simulink model "UAV"  (R2025b)
settings: Solver=ode3  StartTime=0.0  StopTime=inf  FixedStep=Sim.Ts_fisica  RelTol=1e-3
PostLoadFcn:
  | Init
InitFcn:
  | Init
model workspace (MAT data in the model file):
  Mass = 1
undefined symbols (not defined in the file): DiscIntNeverNeededParam, Drone, DWORK0, DWORK1, DWORK10, DWORK11, DWORK12, DWORK13, DWORK14, DWORK15, DWORK16, DWORK17, DWORK18, DWORK19, DWORK2, DWORK20, DWORK21, DWORK22, DWORK23, DWORK24, DWORK3, DWORK4, DWORK5, DWORK6, DWORK7, DWORK8, DWORK9, F, Light, MIL, Sim
libraries: simulink x35, slpidlib x11, vrlib x4, aerolibwind2 x2, sim3dlib x2, uavsim3dlib x2
(part 8 of 8)

== system UAV/Pilot Interface/SIM_Flightstick_HotasX56 /Command Acquisition/Subsystem ==
  In1 : Inport
  Dead Zone{,1..4} (5 alike) : DeadZone  LowerValue=-0.05  UpperValue=0.05
  Demux : Demux  Outputs=5
  Selector : Selector  InputPortWidth=5  IndexOptions=Index vector (dialog)  Indices=[1 2 3 4 5]  OutputSizes=1
  Zero-Order Hold : ZeroOrderHold  SampleTime=1/100
  Roll : Outport
  Pitch : Outport  Port=2
  Yaw : Outport  Port=3
  Cx : Outport  Port=4
  Cy : Outport  Port=5
  wires:
  Demux/5 -> Dead Zone4/1
  Demux/4 -> Dead Zone3/1
  Demux/2 -> Dead Zone1/1
  Demux/3 -> Dead Zone2/1
  Demux/1 -> Dead Zone/1
  In1/1 -> Zero-Order Hold/1
  Selector/1 -> Demux/1
  Zero-Order Hold/1 -> Selector/1
  Dead Zone/1 -> Roll/1
  Dead Zone1/1 -> Pitch/1
  Dead Zone2/1 -> Cx/1
  Dead Zone3/1 -> Cy/1
  Dead Zone4/1 -> Yaw/1

== system UAV/Pilot Interface/SIM_Flightstick_HotasX56 /Command Acquisition/Subsystem1 ==
  In1 : Inport
  Demux1 : Demux  Outputs=14
  Selector : Selector  InputPortWidth=17  IndexOptions=Index vector (dialog)  Indices=[1 2 3 4 5 6 7 8 9 10 11 12 13 14]  OutputSizes=1
  Zero-Order Hold1 : ZeroOrderHold  SampleTime=1/100
  Trigger : Outport
  A : Outport  Port=2
  B : Outport  Port=3
  "C " : Outport  Port=4
  "D " : Outport  Port=5
  Lever : Outport  Port=6
  H1U : Outport  Port=7
  H1R : Outport  Port=8
  H1D : Outport  Port=9
  H1L : Outport  Port=10
  H2U : Outport  Port=11
  H2R : Outport  Port=12
  H2D : Outport  Port=13
  H2L : Outport  Port=14
  wires:
  In1/1 -> Zero-Order Hold1/1
  Selector/1 -> Demux1/1
  Demux1/1 -> Trigger/1
  Demux1/2 -> A/1
  Demux1/3 -> B/1
  Demux1/4 -> "C "/1
  Demux1/5 -> "D "/1
  Demux1/6 -> Lever/1
  Demux1/7 -> H1U/1
  Demux1/8 -> H1R/1
  Demux1/9 -> H1D/1
  Demux1/10 -> H1L/1
  Demux1/11 -> H2U/1
  Demux1/12 -> H2R/1
  Demux1/13 -> H2D/1
  Demux1/14 -> H2L/1
  Zero-Order Hold1/1 -> Selector/1

== system UAV/Pilot Interface/SIM_Flightstick_HotasX56 /Command Acquisition/Subsystem2 ==
  In1 : Inport
  Compare To Constant : simulink/Logic and Bit Operations/Compare To Constant  relop===  const=0  OutDataTypeStr=boolean
  Compare To Constant1 : simulink/Logic and Bit Operations/Compare To Constant  relop===  const=90  OutDataTypeStr=boolean
  Compare To Constant2 : simulink/Logic and Bit Operations/Compare To Constant  relop===  const=180  OutDataTypeStr=boolean
  Compare To Constant3 : simulink/Logic and Bit Operations/Compare To Constant  relop===  const=270  OutDataTypeStr=boolean
  Selector : Selector  InputPortWidth=1  IndexOptions=Index vector (dialog)  Indices=[1]  OutputSizes=1
  Zero-Order Hold2 : ZeroOrderHold  SampleTime=1/100
  POV_U : Outport
  POV_R : Outport  Port=2
  POV_D : Outport  Port=3
  POV_L : Outport  Port=4
  wires:
  In1/1 -> Zero-Order Hold2/1
  Zero-Order Hold2/1 -> Selector/1
  Compare To Constant/1 -> POV_U/1
  Compare To Constant1/1 -> POV_R/1
  Compare To Constant2/1 -> POV_D/1
  Compare To Constant3/1 -> POV_L/1
  Selector/1 -> Compare To Constant3/1, Compare To Constant2/1, Compare To Constant1/1, Compare To Constant/1

== system UAV/Pilot Interface/SIM_Flightstick_HotasX56 /Command Acquisition/Subsystem3 ==
  In1 : Inport
  Dead Zone{,1..7} (8 alike) : DeadZone  LowerValue=-0.05  UpperValue=0.05
  Demux : Demux  Outputs=8
  Selector : Selector  InputPortWidth=8  IndexOptions=Index vector (dialog)  Indices=[1 2 3 4 5 6 7 8]  OutputSizes=1
  Zero-Order Hold : ZeroOrderHold  SampleTime=1/100
  Left TL : Outport
  Right TL : Outport  Port=2
  F : Outport  Port=3
  Cx : Outport  Port=4
  Cy : Outport  Port=5
  G : Outport  Port=6
  RTY 3 : Outport  Port=7
  RTY 4 : Outport  Port=8
  wires:
  Demux/5 -> Dead Zone4/1
  Demux/4 -> Dead Zone3/1
  Demux/2 -> Dead Zone1/1
  Demux/3 -> Dead Zone2/1
  Demux/1 -> Dead Zone/1
  In1/1 -> Zero-Order Hold/1
  Selector/1 -> Demux/1
  Zero-Order Hold/1 -> Selector/1
  Demux/6 -> Dead Zone5/1
  Demux/7 -> Dead Zone6/1
  Demux/8 -> Dead Zone7/1
  Dead Zone1/1 -> Right TL/1
  Dead Zone2/1 -> F/1
  Dead Zone3/1 -> Cx/1
  Dead Zone4/1 -> Cy/1
  Dead Zone5/1 -> G/1
  Dead Zone6/1 -> RTY 3/1
  Dead Zone7/1 -> RTY 4/1
  Dead Zone/1 -> Left TL/1

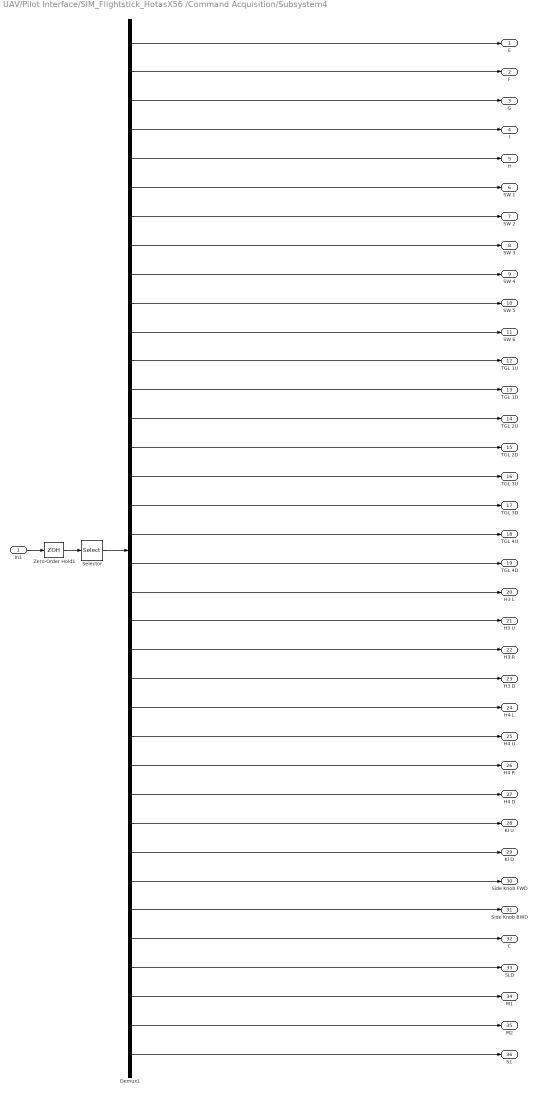
== system UAV/Pilot Interface/SIM_Flightstick_HotasX56 /Command Acquisition/Subsystem4 ==
  In1 : Inport
  Demux1 : Demux  Outputs=36
  Selector : Selector  InputPortWidth=36  IndexOptions=Index vector (dialog)  Indices=[1 2 3 4 5 6 7 8 9 10 11 12 13 14 15 16 17 18 19 20 21 22 23 24 25 26 27 28 29 30 31 32 33 34 35 36]  OutputSizes=1
  Zero-Order Hold1 : ZeroOrderHold  SampleTime=1/100
  E : Outport
  F : Outport  Port=2
  G : Outport  Port=3
  I : Outport  Port=4
  H : Outport  Port=5
  SW 1 : Outport  Port=6
  SW 2 : Outport  Port=7
  SW 3 : Outport  Port=8
  SW 4 : Outport  Port=9
  SW 5 : Outport  Port=10
  SW 6 : Outport  Port=11
  TGL 1U : Outport  Port=12
  TGL 1D : Outport  Port=13
  TGL 2U : Outport  Port=14
  TGL 2D : Outport  Port=15
  TGL 3U : Outport  Port=16
  TGL 3D : Outport  Port=17
  TGL 4U : Outport  Port=18
  TGL 4D : Outport  Port=19
  H3 L : Outport  Port=20
  H3 U : Outport  Port=21
  H3 R : Outport  Port=22
  H3 D : Outport  Port=23
  H4 L : Outport  Port=24
  H4 U : Outport  Port=25
  H4 R : Outport  Port=26
  H4 D : Outport  Port=27
  KI U : Outport  Port=28
  KI D : Outport  Port=29
  Side Knob FWD : Outport  Port=30
  Side Knob BWD : Outport  Port=31
  C : Outport  Port=32
  SLD : Outport  Port=33
  M1 : Outport  Port=34
  M2 : Outport  Port=35
  S1 : Outport  Port=36
  wires:
  Selector/1 -> Demux1/1
  Zero-Order Hold1/1 -> Selector/1
  In1/1 -> Zero-Order Hold1/1
  Demux1/1 -> E/1
  Demux1/2 -> F/1
  Demux1/3 -> G/1
  Demux1/5 -> H/1
  Demux1/6 -> SW 1/1
  Demux1/7 -> SW 2/1
  Demux1/8 -> SW 3/1
  Demux1/9 -> SW 4/1
  Demux1/13 -> TGL 1D/1
  Demux1/14 -> TGL 2U/1
  Demux1/15 -> TGL 2D/1
  Demux1/16 -> TGL 3U/1
  Demux1/17 -> TGL 3D/1
  Demux1/18 -> TGL 4U/1
  Demux1/19 -> TGL 4D/1
  Demux1/20 -> H3 L/1
  Demux1/21 -> H3 U/1
  Demux1/22 -> H3 R/1
  Demux1/23 -> H3 D/1
  Demux1/24 -> H4 L/1
  Demux1/25 -> H4 U/1
  Demux1/26 -> H4 R/1
  Demux1/27 -> H4 D/1
  Demux1/28 -> KI U/1
  Demux1/29 -> KI D/1
  Demux1/30 -> Side Knob FWD/1
  Demux1/31 -> Side Knob BWD/1
  Demux1/32 -> C/1
  Demux1/33 -> SLD/1
  Demux1/34 -> M1/1
  Demux1/35 -> M2/1
  Demux1/36 -> S1/1
  Demux1/4 -> I/1
  Demux1/10 -> SW 5/1
  Demux1/11 -> SW 6/1
  Demux1/12 -> TGL 1U/1

== system UAV/Pilot Interface/SIM_Flightstick_HotasX56 /Flight Data Display/Subsystem ==
  seg : Inport
  Compose String : ComposeString  Format="\"%02d:%02d\""
  Constant : Constant  Value=60
  Data Type Conversion : DataTypeConversion  SaturateOnIntegerOverflow=off  RndMeth=Floor
  Data Type Conversion1 : DataTypeConversion  SaturateOnIntegerOverflow=off  RndMeth=Floor
  Floor : Rounding
  Floor1 : Rounding
  Gain : Gain  Gain=1/60
  Math Function : Math  Operator=mod
  MM:SS : Outport
  wires:
  Constant/1 -> Math Function/2
  Gain/1 -> Floor/1
  Floor1/1 -> Data Type Conversion1/1
  Data Type Conversion/1 -> Compose String/1
  Data Type Conversion1/1 -> Compose String/2
  Math Function/1 -> Floor1/1
  Floor/1 -> Data Type Conversion/1
  seg/1 -> Gain/1, Math Function/1
  Compose String/1 -> MM:SS/1

== system UAV/Vehicle Interface/Real_Hardware_Drivers/Body Dynamics/  ==
  Vb : Inport
  Add3 : Sum  Inputs=+++
  Constant : Constant  Value=0.1
  Demux : Demux  Outputs=3
  Max : MinMax  Function=max  Inputs=2
  Sqrt : Sqrt
  Square : Math  Operator=square  SignedPower=on  RndMeth=Zero
  Square1 : Math  Operator=square  SignedPower=on  RndMeth=Zero
  Square2 : Math  Operator=square  SignedPower=on  RndMeth=Zero
  V : Outport
  wires:
  Square1/1 -> Add3/2
  Square/1 -> Add3/1
  Add3/1 -> Sqrt/1
  Square2/1 -> Add3/3
  Demux/1 -> Square/1
  Demux/2 -> Square1/1
  Demux/3 -> Square2/1
  Vb/1 -> Demux/1
  Constant/1 -> Max/2
  Sqrt/1 -> Max/1
  Max/1 -> V/1

== system UAV/Vehicle Interface/Real_Hardware_Drivers/Body Dynamics/   ==
  Xe : Inport
  Abs : Abs  SaturateOnIntegerOverflow=off
  Constant : Constant  Value=0.5
  Max : MinMax  Function=max  Inputs=2
  Selector : Selector  InputPortWidth=3  IndexOptions=Index vector (dialog)  Indices=[3]  OutputSizes=1
  h : Outport
  wires:
  Selector/1 -> Abs/1
  Xe/1 -> Selector/1
  Constant/1 -> Max/2
  Max/1 -> h/1
  Abs/1 -> Max/1

== system UAV/Vehicle Interface/Real_Hardware_Drivers/Body Dynamics/Dynanic Wind NED ==
  Cos : Trigonometry  Operator=cos
  Cos1 : Trigonometry
  Gain : Gain  Gain=pi/180
  Mux : Mux  Inputs=3
  Product2 : Product
  Product3 : Product
  Wind Dir : Constant  Value=0
  Wind Speed : Constant  Value=0
  Out1 : Outport
  wires:
  Cos/1 -> Product2/2
  Wind Dir/1 -> Gain/1
  Product3/1 -> Mux/2
  Mux/1 -> Out1/1
  Cos1/1 -> Product3/2
  Wind Speed/1 -> Product2/1, Product3/1
  Product2/1 -> Mux/1
  Gain/1 -> Cos/1, Cos1/1

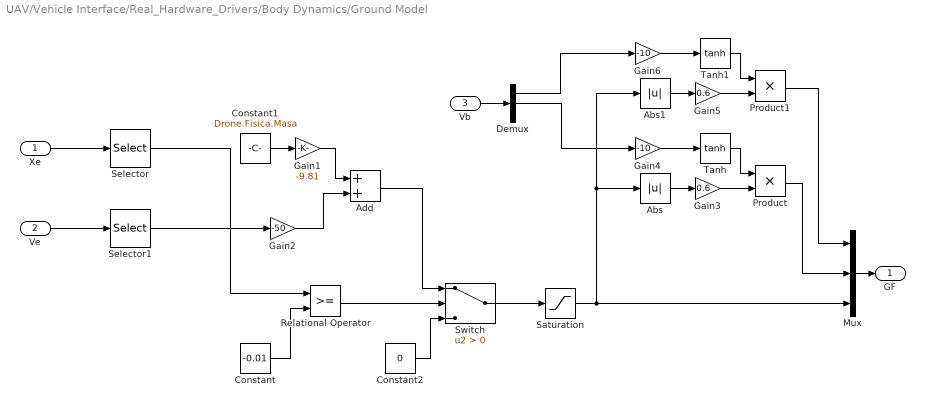
== system UAV/Vehicle Interface/Real_Hardware_Drivers/Body Dynamics/Ground Model ==
  Xe : Inport
  Ve : Inport  Port=2
  Vb : Inport  Port=3
  Abs : Abs  SaturateOnIntegerOverflow=off
  Abs1 : Abs  SaturateOnIntegerOverflow=off
  Add : Sum
  Constant : Constant  Value=-0.01
  Constant1 : Constant  Value=Drone.Fisica.Masa
  Constant2 : Constant  Value=0
  Demux : Demux  Outputs=3
  Gain1 : Gain  Gain=-9.81
  Gain2 : Gain  Gain=-50
  Gain3 : Gain  Gain=0.6
  Gain4 : Gain  Gain=-10
  Gain5 : Gain  Gain=0.6
  Gain6 : Gain  Gain=-10
  Mux : Mux  Inputs=3
  Product : Product
  Product1 : Product
  Relational Operator : RelationalOperator  OutDataTypeStr=boolean  RndMeth=Simplest  InputSameDT=off
  Saturation : Saturate  UpperLimit=0  LowerLimit=-inf
  Selector : Selector  InputPortWidth=3  IndexOptions=Index vector (dialog)  Indices=[3]  OutputSizes=1
  Selector1 : Selector  InputPortWidth=3  IndexOptions=Index vector (dialog)  Indices=[3]  OutputSizes=1
  Switch : Switch  Criteria=u2 > Threshold  SaturateOnIntegerOverflow=off  InputSameDT=off
  Tanh : Trigonometry  Operator=tanh
  Tanh1 : Trigonometry  Operator=tanh
  GF : Outport
  wires:
  Ve/1 -> Selector1/1
  Xe/1 -> Selector/1
  Selector/1 -> Relational Operator/1
  Relational Operator/1 -> Switch/2
  Gain1/1 -> Add/1
  Selector1/1 -> Gain2/1
  Constant/1 -> Relational Operator/2
  Add/1 -> Switch/1
  Constant2/1 -> Switch/3
  Switch/1 -> Saturation/1
  Gain2/1 -> Add/2
  Mux/1 -> GF/1
  Saturation/1 -> Abs/1, Abs1/1, Mux/3
  Abs/1 -> Gain3/1
  Gain4/1 -> Tanh/1
  Gain3/1 -> Product/2
  Tanh/1 -> Product/1
  Gain5/1 -> Product1/2
  Gain6/1 -> Tanh1/1
  Tanh1/1 -> Product1/1
  Abs1/1 -> Gain5/1
  Product1/1 -> Mux/1
  Product/1 -> Mux/2
  Vb/1 -> Demux/1
  Demux/1 -> Gain6/1
  Demux/2 -> Gain4/1
  Constant1/1 -> Gain1/1

== system UAV/Vehicle Interface/Real_Hardware_Drivers/Sensors/Barometer ==
  Xe : Inport
  Band-Limited White Noise : simulink/Sources/Band-Limited White Noise  Cov=Drone.Sensors.Baro.NoisePower  Ts=Sim.Ts_baro  seed=[23341]
  Bias : Bias  Bias=150  SaturateOnIntegerOverflow=off
  Gain : Gain  Gain=-1
  Selector : Selector  InputPortWidth=3  IndexOptions=Index vector (dialog)  Indices=[3]  OutputSizes=1
  Sum : Sum  Inputs=|++
  Zero-Order Hold : ZeroOrderHold  SampleTime=Sim.Ts_baro
  z_m : Outport
  wires:
  Xe/1 -> Selector/1
  Sum/1 -> z_m/1
  Selector/1 -> Gain/1
  Gain/1 -> Bias/1
  Bias/1 -> Zero-Order Hold/1
  Zero-Order Hold/1 -> Sum/1
  Band-Limited White Noise/1 -> Sum/2

== system UAV/Vehicle Interface/Real_Hardware_Drivers/Sensors/GPS ==
  Ve : Inport
  Xe : Inport  Port=2
  Band-Limited White Noise : simulink/Sources/Band-Limited White Noise  Cov=Drone.Sensors.GPS.Pos_NoisePower  Ts=Sim.Ts_gps  seed=[23341]
  Band-Limited White Noise1 : simulink/Sources/Band-Limited White Noise  Cov=Drone.Sensors.GPS.Vel_NoisePower  Ts=Sim.Ts_gps  seed=[23341]
  Scope : Scope
      settings: ActiveDisplayYMinimum=-6.1563901872862452  ActiveDisplayYMaximum=9.5685635864458938  DataLoggingVariableName=ScopeData3
  Selector : Selector  InputPortWidth=3  IndexOptions=Index vector (dialog)  Indices=[1]  OutputSizes=1
  Sum : Sum  Inputs=|++
  Sum1 : Sum  Inputs=|++
  Transport Delay : TransportDelay  DelayTime=0.2
  Transport Delay1 : TransportDelay  DelayTime=0.2
  Zero-Order Hold : ZeroOrderHold  SampleTime=Sim.Ts_gps
  Zero-Order Hold1 : ZeroOrderHold  SampleTime=Sim.Ts_gps
  Ve_m : Outport
  Xe_m : Outport  Port=2
  wires:
  Transport Delay/1 -> Zero-Order Hold1/1
  Transport Delay1/1 -> Zero-Order Hold/1
  Sum/1 -> Selector/1, Ve_m/1
  Sum1/1 -> Xe_m/1
  Zero-Order Hold1/1 -> Sum1/1
  Xe/1 -> Transport Delay/1
  Zero-Order Hold/1 -> Sum/1
  Ve/1 -> Transport Delay1/1
  Band-Limited White Noise/1 -> Sum1/2
  Band-Limited White Noise1/1 -> Sum/2
  Selector/1 -> Scope/1

== system UAV/Vehicle Interface/Real_Hardware_Drivers/Sensors/IMU ==
  DCMbe : Inport
  Vb_gt : Inport  Port=2
  Wb_gt : Inport  Port=3
  Accelerometer : Subsystem
  Gyroscope : Subsystem
  Acc_m : Outport
  Gyro_m : Outport  Port=2
  wires:
  Gyroscope/1(Out1) -> Gyro_m/1
  Wb_gt/1 -> Gyroscope/1(In1)
  Accelerometer/1(Out1) -> Acc_m/1
  Vb_gt/1 -> Accelerometer/1(Vb_gt)
  DCMbe/1 -> Accelerometer/2(DCMbe)

== system UAV/Vehicle Interface/Real_Hardware_Drivers/Sensors/Magnetometer ==
  DCMbe : Inport
  Band-Limited White Noise : simulink/Sources/Band-Limited White Noise  Cov=Drone.Sensors.Mag.NoisePower  Ts=Sim.Ts_mag  seed=[23, 45, 67]
  Bias : Bias  Bias=[0.1; -0.05; 0.05]  SaturateOnIntegerOverflow=off
  Mag_field : Constant  Value=[0.6;0;0.8]
  Product : Product  Multiplication=Matrix(*)
  Sum : Sum  Inputs=|++
  Zero-Order Hold : ZeroOrderHold  SampleTime=Sim.Ts_mag
  Mag_m : Outport
  wires:
  Product/1 -> Bias/1
  Mag_field/1 -> Product/2
  Band-Limited White Noise/1 -> Sum/2
  Zero-Order Hold/1 -> Sum/1
  DCMbe/1 -> Product/1
  Bias/1 -> Zero-Order Hold/1
  Sum/1 -> Mag_m/1

== system UAV/Vehicle Interface/Real_Hardware_Drivers/Visualization/NED to ENU ==
  T_NED : Inport
  R_NED : Inport  Port=2
  Gain4 : Gain  Gain=[0 1 0; 1 0 0; 0 0 -1]  Multiplication=Matrix(K*u) (u vector)
  Gain5 : Gain  Gain=[1 0 0; 0 -1 0; 0 0 -1]  Multiplication=Matrix(K*u) (u vector)
  Gain6 : Gain  Gain=[1,0,0;0,-1,0;0,0,-1]  Multiplication=Matrix(K*u) (u vector)
  Gain7 : Gain  Gain=[0,0,-1;0,-1,0;1,0,0]  Multiplication=Matrix(K*u) (u vector)
  T_ENU : Outport
  R_ENU : Outport  Port=2
  wires:
  R_NED/1 -> Gain7/1
  T_NED/1 -> Gain6/1
  Gain6/1 -> T_ENU/1
  Gain7/1 -> R_ENU/1

== system UAV/Vehicle Interface/Sim_Plant_Model/Body Dynamics/  ==
  Vb : Inport
  Add3 : Sum  Inputs=+++
  Constant : Constant  Value=0.1
  Demux : Demux  Outputs=3
  Max : MinMax  Function=max  Inputs=2
  Sqrt : Sqrt
  Square : Math  Operator=square  SignedPower=on  RndMeth=Zero
  Square1 : Math  Operator=square  SignedPower=on  RndMeth=Zero
  Square2 : Math  Operator=square  SignedPower=on  RndMeth=Zero
  V : Outport
  wires:
  Square1/1 -> Add3/2
  Square/1 -> Add3/1
  Add3/1 -> Sqrt/1
  Square2/1 -> Add3/3
  Demux/1 -> Square/1
  Demux/2 -> Square1/1
  Demux/3 -> Square2/1
  Vb/1 -> Demux/1
  Constant/1 -> Max/2
  Sqrt/1 -> Max/1
  Max/1 -> V/1

== system UAV/Vehicle Interface/Sim_Plant_Model/Body Dynamics/   ==
  Xe : Inport
  Abs : Abs  SaturateOnIntegerOverflow=off
  Constant : Constant  Value=0.5
  Max : MinMax  Function=max  Inputs=2
  Selector : Selector  InputPortWidth=3  IndexOptions=Index vector (dialog)  Indices=[3]  OutputSizes=1
  h : Outport
  wires:
  Selector/1 -> Abs/1
  Xe/1 -> Selector/1
  Constant/1 -> Max/2
  Max/1 -> h/1
  Abs/1 -> Max/1

== system UAV/Vehicle Interface/Sim_Plant_Model/Body Dynamics/Dynanic Wind NED ==
  Cos : Trigonometry  Operator=cos
  Cos1 : Trigonometry
  Gain : Gain  Gain=pi/180
  Mux : Mux  Inputs=3
  Product2 : Product
  Product3 : Product
  Wind Dir : Constant  Value=0
  Wind Speed : Constant  Value=0
  Out1 : Outport
  wires:
  Cos/1 -> Product2/2
  Wind Dir/1 -> Gain/1
  Product3/1 -> Mux/2
  Mux/1 -> Out1/1
  Cos1/1 -> Product3/2
  Wind Speed/1 -> Product2/1, Product3/1
  Product2/1 -> Mux/1
  Gain/1 -> Cos/1, Cos1/1

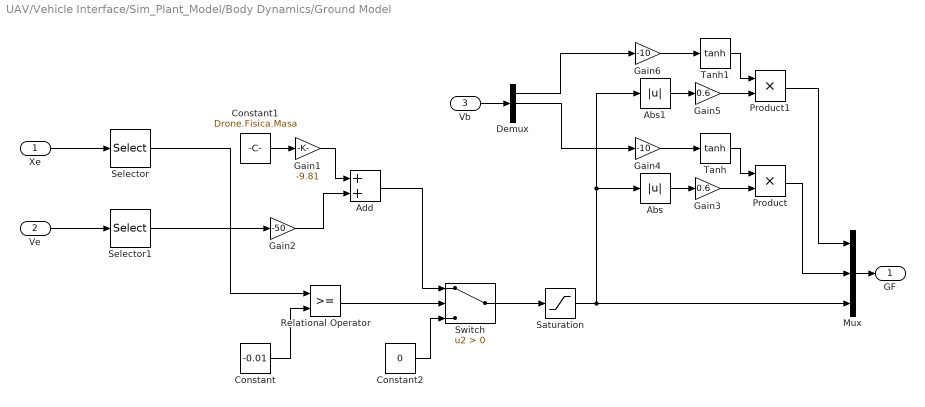
== system UAV/Vehicle Interface/Sim_Plant_Model/Body Dynamics/Ground Model ==
  Xe : Inport
  Ve : Inport  Port=2
  Vb : Inport  Port=3
  Abs : Abs  SaturateOnIntegerOverflow=off
  Abs1 : Abs  SaturateOnIntegerOverflow=off
  Add : Sum
  Constant : Constant  Value=-0.01
  Constant1 : Constant  Value=Drone.Fisica.Masa
  Constant2 : Constant  Value=0
  Demux : Demux  Outputs=3
  Gain1 : Gain  Gain=-9.81
  Gain2 : Gain  Gain=-50
  Gain3 : Gain  Gain=0.6
  Gain4 : Gain  Gain=-10
  Gain5 : Gain  Gain=0.6
  Gain6 : Gain  Gain=-10
  Mux : Mux  Inputs=3
  Product : Product
  Product1 : Product
  Relational Operator : RelationalOperator  OutDataTypeStr=boolean  RndMeth=Simplest  InputSameDT=off
  Saturation : Saturate  UpperLimit=0  LowerLimit=-inf
  Selector : Selector  InputPortWidth=3  IndexOptions=Index vector (dialog)  Indices=[3]  OutputSizes=1
  Selector1 : Selector  InputPortWidth=3  IndexOptions=Index vector (dialog)  Indices=[3]  OutputSizes=1
  Switch : Switch  Criteria=u2 > Threshold  SaturateOnIntegerOverflow=off  InputSameDT=off
  Tanh : Trigonometry  Operator=tanh
  Tanh1 : Trigonometry  Operator=tanh
  GF : Outport
  wires:
  Ve/1 -> Selector1/1
  Xe/1 -> Selector/1
  Selector/1 -> Relational Operator/1
  Relational Operator/1 -> Switch/2
  Gain1/1 -> Add/1
  Selector1/1 -> Gain2/1
  Constant/1 -> Relational Operator/2
  Add/1 -> Switch/1
  Constant2/1 -> Switch/3
  Switch/1 -> Saturation/1
  Gain2/1 -> Add/2
  Mux/1 -> GF/1
  Saturation/1 -> Abs/1, Abs1/1, Mux/3
  Abs/1 -> Gain3/1
  Gain4/1 -> Tanh/1
  Gain3/1 -> Product/2
  Tanh/1 -> Product/1
  Gain5/1 -> Product1/2
  Gain6/1 -> Tanh1/1
  Tanh1/1 -> Product1/1
  Abs1/1 -> Gain5/1
  Product1/1 -> Mux/1
  Product/1 -> Mux/2
  Vb/1 -> Demux/1
  Demux/1 -> Gain6/1
  Demux/2 -> Gain4/1
  Constant1/1 -> Gain1/1

== system UAV/Vehicle Interface/Sim_Plant_Model/Sensors/Barometer ==
  Xe : Inport
  Band-Limited White Noise : simulink/Sources/Band-Limited White Noise  Cov=Drone.Sensors.Baro.NoisePower  Ts=Sim.Ts_baro  seed=[23341]
  Bias : Bias  Bias=150  SaturateOnIntegerOverflow=off
  Gain : Gain  Gain=-1
  Selector : Selector  InputPortWidth=3  IndexOptions=Index vector (dialog)  Indices=[3]  OutputSizes=1
  Sum : Sum  Inputs=|++
  Zero-Order Hold : ZeroOrderHold  SampleTime=Sim.Ts_baro
  z_m : Outport
  wires:
  Xe/1 -> Selector/1
  Sum/1 -> z_m/1
  Selector/1 -> Gain/1
  Gain/1 -> Bias/1
  Bias/1 -> Zero-Order Hold/1
  Zero-Order Hold/1 -> Sum/1
  Band-Limited White Noise/1 -> Sum/2

== system UAV/Vehicle Interface/Sim_Plant_Model/Sensors/GPS ==
  Ve : Inport
  Xe : Inport  Port=2
  Band-Limited White Noise : simulink/Sources/Band-Limited White Noise  Cov=Drone.Sensors.GPS.Pos_NoisePower  Ts=Sim.Ts_gps  seed=[23341]
  Band-Limited White Noise1 : simulink/Sources/Band-Limited White Noise  Cov=Drone.Sensors.GPS.Vel_NoisePower  Ts=Sim.Ts_gps  seed=[23341]
  Scope : Scope
      settings: ActiveDisplayYMinimum=-6.1563901872862452  ActiveDisplayYMaximum=9.5685635864458938  DataLoggingVariableName=ScopeData3
  Selector : Selector  InputPortWidth=3  IndexOptions=Index vector (dialog)  Indices=[1]  OutputSizes=1
  Sum : Sum  Inputs=|++
  Sum1 : Sum  Inputs=|++
  Transport Delay : TransportDelay  DelayTime=0.2
  Transport Delay1 : TransportDelay  DelayTime=0.2
  Zero-Order Hold : ZeroOrderHold  SampleTime=Sim.Ts_gps
  Zero-Order Hold1 : ZeroOrderHold  SampleTime=Sim.Ts_gps
  Ve_m : Outport
  Xe_m : Outport  Port=2
  wires:
  Transport Delay/1 -> Zero-Order Hold1/1
  Transport Delay1/1 -> Zero-Order Hold/1
  Sum/1 -> Selector/1, Ve_m/1
  Sum1/1 -> Xe_m/1
  Zero-Order Hold1/1 -> Sum1/1
  Xe/1 -> Transport Delay/1
  Zero-Order Hold/1 -> Sum/1
  Ve/1 -> Transport Delay1/1
  Band-Limited White Noise/1 -> Sum1/2
  Band-Limited White Noise1/1 -> Sum/2
  Selector/1 -> Scope/1

== system UAV/Vehicle Interface/Sim_Plant_Model/Sensors/IMU ==
  DCMbe : Inport
  Vb_gt : Inport  Port=2
  Wb_gt : Inport  Port=3
  Accelerometer : Subsystem
  Gyroscope : Subsystem
  Acc_m : Outport
  Gyro_m : Outport  Port=2
  wires:
  Gyroscope/1(Out1) -> Gyro_m/1
  Wb_gt/1 -> Gyroscope/1(In1)
  Accelerometer/1(Out1) -> Acc_m/1
  Vb_gt/1 -> Accelerometer/1(Vb_gt)
  DCMbe/1 -> Accelerometer/2(DCMbe)

== system UAV/Vehicle Interface/Sim_Plant_Model/Sensors/Magnetometer ==
  DCMbe : Inport
  Band-Limited White Noise : simulink/Sources/Band-Limited White Noise  Cov=Drone.Sensors.Mag.NoisePower  Ts=Sim.Ts_mag  seed=[23, 45, 67]
  Bias : Bias  Bias=[0.1; -0.05; 0.05]  SaturateOnIntegerOverflow=off
  Mag_field : Constant  Value=[0.6;0;0.8]
  Product : Product  Multiplication=Matrix(*)
  Sum : Sum  Inputs=|++
  Zero-Order Hold : ZeroOrderHold  SampleTime=Sim.Ts_mag
  Mag_m : Outport
  wires:
  Product/1 -> Bias/1
  Mag_field/1 -> Product/2
  Band-Limited White Noise/1 -> Sum/2
  Zero-Order Hold/1 -> Sum/1
  DCMbe/1 -> Product/1
  Bias/1 -> Zero-Order Hold/1
  Sum/1 -> Mag_m/1

== system UAV/Vehicle Interface/Sim_Plant_Model/Visualization/NED to ENU ==
  T_NED : Inport
  R_NED : Inport  Port=2
  Gain4 : Gain  Gain=[0 1 0; 1 0 0; 0 0 -1]  Multiplication=Matrix(K*u) (u vector)
  Gain5 : Gain  Gain=[1 0 0; 0 -1 0; 0 0 -1]  Multiplication=Matrix(K*u) (u vector)
  Gain6 : Gain  Gain=[1,0,0;0,-1,0;0,0,-1]  Multiplication=Matrix(K*u) (u vector)
  Gain7 : Gain  Gain=[0,0,-1;0,-1,0;1,0,0]  Multiplication=Matrix(K*u) (u vector)
  T_ENU : Outport
  R_ENU : Outport  Port=2
  wires:
  R_NED/1 -> Gain7/1
  T_NED/1 -> Gain6/1
  Gain6/1 -> T_ENU/1
  Gain7/1 -> R_ENU/1

== system UAV/Vehicle Interface/Real_Hardware_Drivers/Sensors/IMU/Accelerometer ==
  Vb_gt : Inport
  DCMbe : Inport  Port=2
  Add : Sum  Inputs=+-
  Band-Limited White Noise : simulink/Sources/Band-Limited White Noise  Cov=Drone.Sensors.Accel.NoisePower  Ts=Sim.Ts_imu  seed=[23341]
  Derivative : Derivative
  Product : Product  Multiplication=Matrix(*)
  Sum : Sum  Inputs=|++
  Zero-Order Hold : ZeroOrderHold  SampleTime=Sim.Ts_imu
  g : Constant  Value=[0;0;9.81]
  Out1 : Outport
  wires:
  Vb_gt/1 -> Derivative/1
  g/1 -> Product/2
  DCMbe/1 -> Product/1
  Derivative/1 -> Add/1
  Product/1 -> Add/2
  Add/1 -> Zero-Order Hold/1
  Zero-Order Hold/1 -> Sum/1
  Sum/1 -> Out1/1
  Band-Limited White Noise/1 -> Sum/2

== system UAV/Vehicle Interface/Real_Hardware_Drivers/Sensors/IMU/Gyroscope ==
  In1 : Inport
  Band-Limited White Noise : simulink/Sources/Band-Limited White Noise  Cov=Drone.Sensors.Gyro.NoisePower  Ts=Sim.Ts_imu  seed=[23341]
  Bias : Bias  Bias=[0.01, -0.01, 0.005]  SaturateOnIntegerOverflow=off
  Ramp : simulink/Sources/Ramp  slope=[0.00006, 0.00006, 0.00003]  start=5  InitialOutput=0
  Sum : Sum  Inputs=|++
  Sum1 : Sum  Inputs=|++
  Zero-Order Hold : ZeroOrderHold  SampleTime=Sim.Ts_imu
  Out1 : Outport
  wires:
  Band-Limited White Noise/1 -> Sum/2
  Sum1/1 -> Zero-Order Hold/1
  Zero-Order Hold/1 -> Sum/1
  Sum/1 -> Out1/1
  In1/1 -> Bias/1
  Bias/1 -> Sum1/1
  Ramp/1 -> Sum1/2

== system UAV/Vehicle Interface/Sim_Plant_Model/Sensors/IMU/Accelerometer ==
  Vb_gt : Inport
  DCMbe : Inport  Port=2
  Add : Sum  Inputs=+-
  Band-Limited White Noise : simulink/Sources/Band-Limited White Noise  Cov=Drone.Sensors.Accel.NoisePower  Ts=Sim.Ts_imu  seed=[23341]
  Derivative : Derivative
  Product : Product  Multiplication=Matrix(*)
  Sum : Sum  Inputs=|++
  Zero-Order Hold : ZeroOrderHold  SampleTime=Sim.Ts_imu
  g : Constant  Value=[0;0;9.81]
  Out1 : Outport
  wires:
  Vb_gt/1 -> Derivative/1
  g/1 -> Product/2
  DCMbe/1 -> Product/1
  Derivative/1 -> Add/1
  Product/1 -> Add/2
  Add/1 -> Zero-Order Hold/1
  Zero-Order Hold/1 -> Sum/1
  Sum/1 -> Out1/1
  Band-Limited White Noise/1 -> Sum/2

== system UAV/Vehicle Interface/Sim_Plant_Model/Sensors/IMU/Gyroscope ==
  In1 : Inport
  Band-Limited White Noise : simulink/Sources/Band-Limited White Noise  Cov=Drone.Sensors.Gyro.NoisePower  Ts=Sim.Ts_imu  seed=[23341]
  Bias : Bias  Bias=[0.01, -0.01, 0.005]  SaturateOnIntegerOverflow=off
  Ramp : simulink/Sources/Ramp  slope=[0.00006, 0.00006, 0.00003]  start=5  InitialOutput=0
  Sum : Sum  Inputs=|++
  Sum1 : Sum  Inputs=|++
  Zero-Order Hold : ZeroOrderHold  SampleTime=Sim.Ts_imu
  Out1 : Outport
  wires:
  Band-Limited White Noise/1 -> Sum/2
  Sum1/1 -> Zero-Order Hold/1
  Zero-Order Hold/1 -> Sum/1
  Sum/1 -> Out1/1
  In1/1 -> Bias/1
  Bias/1 -> Sum1/1
  Ramp/1 -> Sum1/2

== matlab function UAV/Flight Controller Software/Flight Controller Software MIL/State Estimator/MATLAB Function2 ==
  data: bias_est output; raw_accel_vec input; gyro_rates input; mag_body input; system_ready input; angle_est output; DCM_be output
function [bias_est, angle_est, DCM_be] = Attitude_Estimator(raw_accel_vec, gyro_rates, mag_body, system_ready)
% ATTITUDE_ESTIMATOR  Estimador de Orientación (AHRS) basado en EKF.
%
%   Implementa un Filtro de Kalman Extendido (EKF) de 6 estados para fusión sensorial.
%   Combina giroscopio (predicción), acelerómetro (corrección Roll/Pitch) y 
%   magnetómetro (corrección Yaw con compensación de inclinación).
%
%   INPUTS:
%       raw_accel_vec : [ax; ay; az] en m/s^2 (Body Frame)
%       gyro_rates    : [p; q; r] en rad/s (Body Frame)
%       mag_body      : [mx; my; mz] gauss/uT (Body Frame)
%       system_ready  : Flag booleano (0=Calibración, 1=Vuelo)
%
%   OUTPUTS:
%       angle_est     : [Roll; Pitch; Yaw] en radianes (NED Frame)
%       DCM_be        : Matriz de Rotación 3x3 (Body -> Earth)
%       bias_est      : [bp; bq; br] Bias estimado del giroscopio

    % --- SYSTEM CONFIGURATION ---
    Ts = 0.001;  % Sample Time [s] (1 kHz)
    
    persistent x P Q R_acc R_mag ...
               accel_filtrado_prev is_frozen bias_captured ...
               calib_sum calib_count calib_bias_mem ...
               mag_offset_sum mag_yaw_offset
               
    % --- INITIALIZATION (First Run) ---
    if isempty(x)
        x = zeros(6, 1); 
        P = diag([0.001, 0.0001, 0.001, 0.0001, 0.001, 0.0001]);
        Q = diag([0.0001, 1e-6, 0.0001, 1e-6, 0.0001, 1e-5]); 
        R_acc = diag([500, 500]); 
        R_mag = 5; 
        
        accel_filtrado_prev = [0; 0; 0];
        is_frozen       = false; 
        bias_captured   = false;   
        calib_sum       = [0; 0; 0]; 
        calib_count     = 0; 
        calib_bias_mem  = [0; 0; 0];
        mag_offset_sum  = 0; 
        mag_yaw_offset  = 0;
    end
    
    % =========================================================================
    % 1. STATIC CALIBRATION & BIAS INITIALIZATION
    % =========================================================================
    if system_ready == 0
        if bias_captured
            calib_sum = [0;0;0]; calib_count=0; bias_captured=false; mag_offset_sum=0; 
        end
        
        calib_sum = calib_sum + gyro_rates;
        
        mx = mag_body(1); my = mag_body(2);
        current_yaw_sample = -atan2(my, mx); 
        mag_offset_sum = mag_offset_sum + current_yaw_sample;
        
        calib_count = calib_count + 1;
        calib_bias_mem = calib_sum / calib_count; 
        mag_yaw_offset = mag_offset_sum / calib_count;
        
        angle_est   = [0; 0; 0]; 
        bias_est    = [0; 0; 0]; 
        DCM_be      = eye(3); 
        return; 
    end
    
    if ~bias_captured
        x(2) = calib_bias_mem(1); 
        x(4) = calib_bias_mem(2); 
        x(6) = calib_bias_mem(3); 
        bias_captured = true; 
    end
    
    % =========================================================================
    % 2. PREDICTION STEP (Time Update)
    % =========================================================================
    p = gyro_rates(1); 
    q = gyro_rates(2); 
    r_corrected = gyro_rates(3) - x(6); 
    
    phi   = x(1); 
    theta = x(3); 
    tt = tan(theta); 
    ct = cos(theta);
    if abs(ct) < 0.01, ct = 0.01; end 
    
    dot_phi   = p + (q * sin(phi) + r_corrected * cos(phi)) * tt;
    dot_theta = q * cos(phi) - r_corrected * sin(phi);
    dot_psi   = (q * sin(phi) + r_corrected * cos(phi)) / ct;
    
    u = [dot_phi; dot_theta; dot_psi];
    
    F = eye(6);
    F(1,2) = -Ts; F(3,4) = -Ts; F(5,6) = -Ts;
    
    G = zeros(6, 3);
    G(1,1) = Ts; G(3,2) = Ts; G(5,3) = Ts;
    
    x_pred = F * x + G * u; 
    P_pred = F * P * F' + Q;
    
    % =========================================================================
    % 3. CORRECTION STEP: ACCELEROMETER (Roll/Pitch)
    % =========================================================================
    acc_corrected = raw_accel_vec; 
    alpha = 0.1; 
    accel_filtrado = (acc_corrected * alpha) + (accel_filtrado_prev * (1 - alpha));
    accel_filtrado_prev = accel_filtrado;
    
    acc_mag = norm(accel_filtrado);
    
    % Lógica de rechazo de aceleraciones dinámicas
    if abs(acc_mag - 9.81) > 0.6
        is_frozen = true;   
    elseif abs(acc_mag - 9.81) < 0.5
        is_frozen = false;  
    end
    
    if is_frozen
        x_post_acc = x_pred; 
        P_post_acc = P_pred;
    else
        ax = -accel_filtrado(1); ay = -accel_filtrado(2); az = -accel_filtrado(3);
        phi_acc   = atan2(ay, az);
        theta_acc = atan2(-ax, sqrt(ay^2 + az^2));
        
        H_acc = zeros(2, 6); 
        H_acc(1,1) = 1; H_acc(2,3) = 1;
        
        y_acc = [phi_acc; theta_acc] - H_acc * x_pred;
        S_acc = H_acc * P_pred * H_acc' + R_acc;
        K_acc = P_pred * H_acc' / S_acc;
        
        x_post_acc = x_pred + K_acc * y_acc;
        P_post_acc = (eye(6) - K_acc * H_acc) * P_pred;
    end
    
    % =========================================================================
    % 4. CORRECTION STEP: MAGNETOMETER (Yaw)
    % =========================================================================
    phi_est   = x_post_acc(1);
    theta_est = x_post_acc(3);
    mx = mag_body(1); my = mag_body(2); mz = mag_body(3);
    
    Xh = mx * cos(theta_est) + my * sin(phi_est) * sin(theta_est) + mz * cos(phi_est) * sin(theta_est);
    Yh = my * cos(phi_est) - mz * sin(phi_est);
    
    psi_mag_raw = -atan2(Yh, Xh); 
    psi_mag_corrected = psi_mag_raw - mag_yaw_offset;
    
    innov = psi_mag_corrected - x_post_acc(5);
    while innov > pi,  innov = innov - 2*pi; end
    while innov < -pi, innov = innov + 2*pi; end
    
    H_mag = zeros(1, 6); 
    H_mag(1,5) = 1; 
    
    S_mag = H_mag * P_post_acc * H_mag' + R_mag;
    K_mag = P_post_acc * H_mag' / S_mag;
    
    x_final = x_post_acc + K_mag * innov;
    P_final = (eye(6) - K_mag * H_mag) * P_post_acc;
    
    % =========================================================================
    % 5. OUTPUT GENERATION
    % =========================================================================
    x = x_final;
    P = P_final;
    
    psi_out = x(5);
    while psi_out > pi,  psi_out = psi_out - 2*pi; end
    while psi_out < -pi, psi_out = psi_out + 2*pi; end
    
    angle_est   = [x(1); x(3); psi_out]; 
    bias_est    = [x(2); x(4); x(6)]; 
    
    DCM_be = angle2dcm(psi_out, x(3), x(1), 'ZYX')';
end

== matlab function UAV/Flight Controller Software/Flight Controller Software MIL/Telemetry/MATLAB Function ==
  data: yaw_rad input; heading output
function heading = fcn(yaw_rad)
    deg = yaw_rad * (180/pi);
    if deg < 0
        heading = deg + 360;
    else
        heading = deg;
    end
end

== stateflow chart UAV/Flight Controller Software/Flight Controller Software MIL/Flight Supervisor/Main_Logic ==
  state MODE_MANAGER [parallel]
    settings: executionOrder=3
    state ACRO
      entry: Mode_Out = 3;
    state STAB
      entry: Mode_Out = 2;
    state GPS
      entry: Mode_Out = 1;
    (default) -> ACRO
    STAB -> ACRO [order 1] : [Mode_In >= 3 || Mode_In < 1]
    ACRO -> STAB [order 1] : [Mode_In == 2]
    ACRO -> GPS [order 2] : [Mode_In == 1]
    GPS -> ACRO [order 1] : [Mode_In >= 3 || Mode_In < 1]
    GPS -> STAB [order 2] : [Mode_In == 2]
    STAB -> GPS [order 2] : [Mode_In == 1]
  state FLIGHT_LOGIC [parallel]
    settings: executionOrder=1
    state OFFLINE
      entry:
      Status_ID = 1;
    state INIT
      entry:
      Status_ID = 2;
    state REJECTED
      entry:
      Status_ID = 5; % 5 = Imagen Naranja
    state DISARMED
      entry:
      Motors_Enable = 0
      Status_ID = 3; % 3 = Imagen Verde
    state ARMED
      entry:
      Motors_Enable = 1
      Status_ID = 4; % 4 = Imagen Roja ARMED
    REJECTED -> OFFLINE [order 1] : [Battery_SW < 10.4] {after(0.5, sec)}
    (default) -> OFFLINE
    INIT -> REJECTED [order 2] : [Arm_SW == 1]
    OFFLINE -> INIT : [Battery_SW > 14]
    INIT -> OFFLINE [order 1] : [Battery_SW < 10.4] {after(1, sec)}
    REJECTED -> INIT [order 2] : [Arm_SW == 0]
    DISARMED -> REJECTED [order 3] : [Arm_SW == 1 && Throttle >= 0.05]
    INIT -> DISARMED [order 3] : [is_ready == 1]
    ARMED -> OFFLINE [order 2] : [Battery_SW < 10.4] {after(1, sec)}
    DISARMED -> OFFLINE [order 1] : [Battery_SW < 10.4] {after(1, sec)}
    DISARMED -> ARMED [order 2] : [Arm_SW == 1 && Throttle < 0.05]
    ARMED -> DISARMED [order 1] : [Arm_SW == 0]
  state POWER_SYSTEM [parallel]
    settings: executionOrder=2
    state POWER_OFF
      entry: is_ready = 0; Motors_Enable = 0;
    state CALIBRATING
      entry: is_ready = 0;
    state POWER_OK
      entry: is_ready = 1;
    (default) -> POWER_OFF
    POWER_OFF -> CALIBRATING : [Battery_SW > 14]
    CALIBRATING -> POWER_OFF [order 1] : [Battery_SW < 10.4] {after(1, sec)}
    POWER_OK -> POWER_OFF : [Battery_SW < 10.4] {after(1, sec)}
    CALIBRATING -> POWER_OK [order 2] : after(3, sec)
  data: Mode_In input; Arm_SW input; Battery_SW input; Status_ID output; Mode_Out output; Motors_Enable output; is_ready local; Throttle input

== matlab function UAV/Flight Controller Software/Flight Controller Software MIL/State Estimator/MATLAB Function ==
  data: acc_body input; pos_ned output; DCM_be input; gps_pos input; gps_vel input; baro_alt input; system_ready input; vel_ned output
function [pos_ned, vel_ned] = Position_Estimator(acc_body, DCM_be, gps_pos, gps_vel, baro_alt, system_ready)
% POSITION_ESTIMATOR  Estimador de Posición y Velocidad (INS/GPS)
%
%   Fusiona datos de Acelerómetro (IMU), GPS y Barómetro usando un EKF.
%   El sistema utiliza un marco de referencia NED (North-East-Down).
%   Recibe la orientación (DCM) calculada externamente para optimizar recursos.
%
%   INPUTS:
%       acc_body     : [ax; ay; az] Aceleración en m/s^2 (Body Frame)
%       DCM_be       : Matriz de Rotación 3x3 (Body -> Earth)
%       gps_pos      : [Lat; Lon; Alt] o [N; E; D] según configuración (m)
%       gps_vel      : [VelN; VelE] Velocidad GPS en m/s
%       baro_alt     : Altura barométrica [m] (Positivo hacia arriba)
%       system_ready : Flag de estado (0=Calibración, 1=Vuelo)
%
%   OUTPUTS:
%       pos_ned      : [Pn; Pe; Pd] Posición estimada [m]
%       vel_ned      : [Vn; Ve; Vd] Velocidad estimada [m/s]

    % --- SYSTEM CONFIGURATION ---
    Ts = 0.02;  % Tiempo de muestreo (50 Hz) - GPS suele ser más lento
    
    persistent x P Q R_base ...
               baro_offset calib_baro_sum calib_count ...
               initialized prev_gps_pos acc_lp
    
    % --- INITIALIZATION (First Run) ---
    if isempty(x)
        % Vector de Estado: [PosN, PosE, PosD, VelN, VelE, VelD]
        x = zeros(6,1); 
        P = eye(6);
        
        % Q: Process Noise (Confianza en la física newtoniana)
        % q_pos: Baja incertidumbre en posición (no hay teletransportación)
        % q_vel: Mayor incertidumbre en velocidad (viento, ráfagas)
        q_pos = 0.0001; 
        q_vel = 0.25;   
        Q = diag([q_pos, q_pos, q_pos, q_vel, q_vel, q_vel].^2);
        
        % R: Measurement Noise (Desviación Estándar de sensores)
        sig_gps_pos = 3.0;  % Precisión GPS ~3 metros
        sig_baro_z  = 4.0;  % Barómetro ruidoso (filtrado agresivo)
        sig_gps_vel = 0.5;  % Precisión Velocidad GPS ~0.5 m/s
        
        % Matriz R Base (se seleccionará dinámicamente según disponibilidad)
        R_base = diag([sig_gps_pos, sig_gps_pos, sig_baro_z, sig_gps_vel, sig_gps_vel].^2);
        
        % Variables de calibración
        baro_offset     = 0;
        calib_baro_sum  = 0;
        calib_count     = 0;
        
        initialized     = false;
        prev_gps_pos    = [0;0;0];
        acc_lp          = [0;0;0]; 
    end
    
    % =========================================================================
    % 1. STATIC CALIBRATION & RESET (Ground Mode)
    % =========================================================================
    if system_ready == 0
        % Acumulamos lecturas del barómetro para encontrar el "Cero Local"
        calib_baro_sum = calib_baro_sum + baro_alt;
        calib_count = calib_count + 1;
        
        baro_offset = calib_baro_sum / calib_count;
        initialized = true;
        
        % Hard Reset del estado físico
        % Asumimos posición GPS actual como verdadera y velocidad cero
        x(1:2) = gps_pos(1:2); % Norte, Este
        x(3)   = 0;            % Abajo (Altura 0 relativa)
        x(4:6) = [0;0;0];      % Velocidades a 0
        
        prev_gps_pos = gps_pos;
        acc_lp       = acc_body; 
        
        pos_ned = x(1:3);
        vel_ned = x(4:6);
        return;
    end
    
    % =========================================================================
    % 2. PRE-PROCESSING (Body Frame)
    % =========================================================================
    % Filtro Paso Bajo (LPF) en acelerómetro para eliminar ruido de motor
    alpha_acc = 0.1; 
    acc_lp = acc_lp * (1 - alpha_acc) + acc_body * alpha_acc;
    
    % =========================================================================
    % 3. ROTATION & GRAVITY COMPENSATION
    % =========================================================================
    % Rotar aceleración del cuerpo al mundo usando la matriz entrante (DCM)
    acc_earth = DCM_be * acc_lp;
    
    % Compensar gravedad (Restar 1G en el eje Z)
    % En sistema NED: La gravedad es +9.81 m/s^2 (Hacia abajo).
    % El acelerómetro mide -9.81 en reposo. Sumamos para cancelar.
    acc_inertial_ned = acc_earth + [0; 0; 9.81]; 
    
    % =========================================================================
    % 4. PREDICTION STEP (Time Update)
    % =========================================================================
    % Modelo de arrastre lineal (Drag) para evitar velocidad infinita
    k_drag = 0.05 * Ts; 
    
    % Matriz de Transición de Estado (F)
    % Pos = Pos + Vel*Ts
    % Vel = Vel * (1 - Drag) + Acc*Ts
    F = eye(6);
    F(1,4) = Ts; F(2,5) = Ts; F(3,6) = Ts; 
    F(4,4) = 1 - k_drag;
    F(5,5) = 1 - k_drag;
    F(6,6) = 1 - k_drag;
    
    % Matriz de Control (G)
    G = [0.5*Ts^2*eye(3); 
             Ts*eye(3)];
         
    x_pred = F * x + G * acc_inertial_ned;
    P_pred = F * P * F' + Q;
    
    % =========================================================================
    % 5. CORRECTION STEP (Measurement Update)
    % =========================================================================
    
    % Preparar medida Barométrica (Invertir signo para NED: Abajo es positivo)
    z_baro_ned = -1 * (baro_alt - baro_offset);
    
    % Detectar si el GPS trajo datos nuevos (es asíncrono)
    is_new_gps = any(gps_pos ~= prev_gps_pos);
    
    if is_new_gps
        % --- CASO A: Fusión Completa (GPS + Barómetro) ---
        prev_gps_pos = gps_pos;
        
        z_meas = [gps_pos(1); gps_pos(2); z_baro_ned; gps_vel(1); gps_vel(2)];
        
        H = zeros(5, 6);
        H(1,1) = 1; H(2,2) = 1; H(3,3) = 1; % Pos N, E, D
        H(4,4) = 1; H(5,5) = 1;             % Vel N, E
        
        R_curr = R_base;
        
    else
        % --- CASO B: Corrección Parcial (Solo Barómetro) ---
        z_meas = z_baro_ned;
        
        H = zeros(1, 6);
        H(1,3) = 1; % Solo observamos estado 3 (Pos D)
        
        R_curr = R_base(3,3); 
    end
    
    % --- Actualización de Kalman (Forma de Joseph para estabilidad) ---
    y = z_meas - H * x_pred;       % Innovación (Medición - Predicción)
    S = H * P_pred * H' + R_curr;  % Covarianza de la Innovación
    K = (P_pred * H') / S;         % Ganancia de Kalman
    
    x = x_pred + K * y;            % Estado Corregido
    
    % Actualización de la Covarianza
    I = eye(6);
    P = (I - K * H) * P_pred * (I - K * H)' + K * R_curr * K';
    
    % =========================================================================
    % 6. OUTPUT GENERATION
    % =========================================================================
    pos_ned = x(1:3);
    vel_ned = x(4:6);
end
